simulink model "NatersV4_cleanV2"  (R2016a)
settings: Solver=FixedStepAuto  StartTime=1  StopTime=12*24*3  FixedStep=1  RelTol=1e-3
InitFcn:
  | %open the initialization function as a structure s
  | clear all
  | model = 'NatersV4_cleanV2';
  | s = system_init(model);
  | clear ans
  | 
  | % time vector
  | t=s.t;
  | t_step = t(2)-t(1);
  | time_u = s.time(1);
  | sample_time = s.sample_time;
  | 
  | % declare parameters
  | Text_D = s.Design(1);
  | Tin_D = s.Design(2);
  | Ts_D = s.Design(3);
  | Tr_D = s.Design(4);
  | Qdot_dem = s.Qdot_dem;
  | L_ini= s.L_ini;
  | 
  | Ab_c = s.Ab_c;
  | Bb_c = s.Bb_c;
  | Tin_sp = s.Tin_sp.signals.values;
  | Text = s.Text.signals.values;
  | Rad_90 = s.rad_90.signals.values;
  | 
  | % k parameters for heat pump model
  | K = s.k;
undefined symbols (not defined in the file or in its folder): DiscIntNeverNeededParam
libraries: simulink x20, carnot x2, dspsigops x1
(part 2 of 2)

== system NatersV4_cleanV2/Heat pump subsystem/cold side/Subsystem ==
  Tcold_out : Inport
  Abs : Abs
  Add : Sum  Inputs=-+
  Constant : Constant  Value=4
  PID Controller : simulink/Continuous/PID Controller  Controller=P  TimeDomain=Discrete-time  SampleTime=-1  IntegratorMethod=Forward Euler  FilterMethod=Forward Euler  Form=Parallel  UseFilter=on  ControllerParametersSource=internal  P=-0.5  I=1  D=0  N=100  InitialConditionSource=internal  InitialConditionForIntegrator=0  InitialConditionForFilter=0  ExternalReset=none  ZeroCross=off  LimitOutput=on  UpperSaturationLimit=1  LowerSaturationLimit=0  LinearizeAsGain=off  AntiWindupMode=none  Kb=1  TrackingMode=off  Kt=1  PParamMin=[]  PParamMax=[]  IParamMin=[]  IParamMax=[]  DParamMin=[]  DParamMax=[]  NParamMin=[]  NParamMax=[]  KbParamMin=[]  KbParamMax=[]  KtParamMin=[]  KtParamMax=[]  POutMin=[]  POutMax=[]  IOutMin=[]  IOutMax=[]  DOutMin=[]  DOutMax=[]  NOutMin=[]  NOutMax=[]  KbOutMin=[]  KbOutMax=[]  KtOutMin=[]  KtOutMax=[]  IntegratorOutMin=[]  IntegratorOutMax=[]  FilterOutMin=[]  FilterOutMax=[]  SumOutMin=[]  SumOutMax=[]  SumI1OutMin=[]  SumI1OutMax=[]  SumI2OutMin=[]  SumI2OutMax=[]  SumI3OutMin=[]  SumI3OutMax=[]  SumDOutMin=[]  SumDOutMax=[]  SaturationOutMin=[]  SaturationOutMax=[]  IntegratorContinuousStateAttributes=''  IntegratorStateMustResolveToSignalObject=off  IntegratorRTWStateStorageClass=Auto  FilterContinuousStateAttributes=''  FilterStateMustResolveToSignalObject=off  FilterRTWStateStorageClass=Auto  DifferentiatorICPrevScaledInput=0  DifferentiatorOutMin=[]  DifferentiatorOutMax=[]
  PID Controller1 : simulink/Continuous/PID Controller  Controller=PI  TimeDomain=Discrete-time  SampleTime=-1  IntegratorMethod=Backward Euler  FilterMethod=Forward Euler  Form=Parallel  UseFilter=on  ControllerParametersSource=internal  P=-0.8  I=-0.2/(60*sample_time)  D=0  N=100  InitialConditionSource=internal  InitialConditionForIntegrator=0  InitialConditionForFilter=0  ExternalReset=none  ZeroCross=off  LimitOutput=on  UpperSaturationLimit=1  LowerSaturationLimit=0  LinearizeAsGain=off  AntiWindupMode=back-calculation  Kb=1  TrackingMode=off  Kt=1  PParamMin=[]  PParamMax=[]  IParamMin=[]  IParamMax=[]  DParamMin=[]  DParamMax=[]  NParamMin=[]  NParamMax=[]  KbParamMin=[]  KbParamMax=[]  KtParamMin=[]  KtParamMax=[]  POutMin=[]  POutMax=[]  IOutMin=[]  IOutMax=[]  DOutMin=[]  DOutMax=[]  NOutMin=[]  NOutMax=[]  KbOutMin=[]  KbOutMax=[]  KtOutMin=[]  KtOutMax=[]  IntegratorOutMin=[]  IntegratorOutMax=[]  FilterOutMin=[]  FilterOutMax=[]  SumOutMin=[]  SumOutMax=[]  SumI1OutMin=[]  SumI1OutMax=[]  SumI2OutMin=[]  SumI2OutMax=[]  SumI3OutMin=[]  SumI3OutMax=[]  SumDOutMin=[]  SumDOutMax=[]  SaturationOutMin=[]  SaturationOutMax=[]  IntegratorContinuousStateAttributes=''  IntegratorStateMustResolveToSignalObject=off  IntegratorRTWStateStorageClass=Auto  FilterContinuousStateAttributes=''  FilterStateMustResolveToSignalObject=off  FilterRTWStateStorageClass=Auto  DifferentiatorICPrevScaledInput=0  DifferentiatorOutMin=[]  DifferentiatorOutMax=[]
  Saturation : Saturate  UpperLimit=1  LowerLimit=0  ZeroCross=off
  Scope{,1,3..4} (4 alike) : Scope
  Switch : Switch  Threshold=1.5
  control : Outport
  wires:
  Tcold_out/1 -> Add/1
  Add/1 -> Scope1/1, PID Controller/1, PID Controller1/1, Abs/1
  Abs/1 -> Switch/2
  PID Controller/1 -> Scope4/1, Switch/1
  PID Controller1/1 -> Switch/3, Scope3/1
  Switch/1 -> Saturation/1
  Constant/1 -> Add/2
  Saturation/1 -> control/1, Scope/1

== system NatersV4_cleanV2/Subsystem/Flow_Mixer_basic/Mix_T_Mdot ==
  THB1 : Inport
  THB2 : Inport  Port=2
  Add : Sum
  MATLAB Function : MATLAB Function  TreatAsAtomicUnit=on
  Scope : Scope
  Scope1 : Scope
  Selector1 : Selector  InputPortWidth=2  IndexOptions=Index vector (dialog)  Indices=[2]  OutputSizes=1
  Selector3 : Selector  InputPortWidth=2  IndexOptions=Index vector (dialog)  Indices=[2]  OutputSizes=1
  T : Outport
  mdot : Outport  Port=2
  wires:
  Add/1 -> mdot/1
  Selector1/1 -> Scope1/1, Add/2
  MATLAB Function/1(T_mix) -> T/1  "T"
  THB1/1 -> MATLAB Function/1(Flow_h), Selector3/1
  THB2/1 -> MATLAB Function/2(Flow_c), Selector1/1
  Selector3/1 -> Scope/1, Add/1

== matlab function NatersV4_cleanV2/Building subsystem/MATLAB Function ==
  data: Tb_in input size=[3 1]; Text input; Gin input; Psol input; Tb_out output size=[3 1]; Tws input; flow_fraction input; t_step parameter; time_u parameter; Qdem output size=1
function [Tb_out, Qdem]  = Simulate_building_dynamics(Tb_in , Text, Gin, Psol, Tws, flow_fraction,t_step, time_u)
%#codegen
% Twr   : Return temperature of the heating system
% Tf    : Temperature of floor
% Tr    : Temperature of the room

% state matrix x = [Twr, Tf, Tin]';
% input matrix u = [Text, Tws, Gin, Psol]'

[Ab_d, Bb_d,K_fr, K_wf,K_ra, C_wr, mc_f, thermal_capacity_flow] = get_state_input_mat_building(flow_fraction,t_step, time_u);

% F, L,
%Tws = 35;

%Tb_out = Ab_d * Tb_in + Bb_d * [Text; Qsup; Gin; Psol];
Tb_out = Ab_d * Tb_in + Bb_d * [Text; Tws; Gin; Psol];
%Qdem = K_fr * (Tb_out(2)-Tb_out(3));

% Qdem2 = K_fr * (Tb_in(1)-Tb_in(2));
Qdem = K_ra * (Tb_in(3)-Text)-Psol-Gin;
%Qdem = K_wf * (Tb_out(1)-Tb_out(2));
%Qsup = FH_st * mc_w * (Tws-Tb_out(1));
% Qsup = K_wf * (Tb_out(1)-Tb_out(2));
% Qin = mc_f * (Tb_in(2)-Tb_out(2))/(60/time_u*60);
% test = (Qdem + Qsup) - Qin;


function [Ab_d, Bb_d, K_fr,K_wf,K_ra, C_return, C_floor, thermal_capacity_flow, Qdot, facHP, nb] = get_state_input_mat_building(floor_heating_flow_fraction, t_step, time_u)

% Create the state matrix and the input matrix for the building system

% state vector for the building
% x_b = [Twr, Tf, Tin]'

% input vector for the building
% u_b = [Text, Tws, Qaux]



[C_return, C_floor, C_room, thermal_capacity_flow, K_wf, K_fr, K_ra, cp_w, Qdot] = get_param_building();
%mw_dot = thermal_capacity_flow * floor_heating_flow_fraction;
mw_dot = floor_heating_flow_fraction;

A = [...
[ -(K_wf + cp_w*mw_dot)/C_return,          K_wf/C_return,                     0];
[                   K_wf/C_floor, -(K_fr + K_wf)/C_floor,          K_fr/C_floor];
[                              0,            K_fr/C_room, -(K_fr + K_ra)/C_room] ...
];

B = [...
[           0, (cp_w*mw_dot)/C_return,        0,        0];
[           0,                      0,        0,        0];
[ K_ra/C_room,                      0, 1/C_room, 1/C_room] ...
];

if time_u == 24
    % time_unit = 'h';
    A = A.*3600;
    B = B.*3600;
elseif time_u == 4 % 1/4h
    A = A.*60*15;
    B = B.*60*15;
elseif time_u == 12 % 5 min
    A = A.*60*5;
    B = B.*60*5;
elseif time_u == 60 % 1 min
    A = A.*60;
    B = B.*60;  
elseif time_u == 60 % 1 min
    A = A.*1;
    B = B.*1;    
end

Ab_d = expm(t_step*A);
Bb_d = A\(Ab_d-eye(size(A, 1)))*B;


function [C_wr, mc_f, C_r, mdot_d_w, K_wf, K_fr, K_ra, cp_w, Q_D] = get_param_building()
%GET_PARAM_BUILDING returns the parameters of the selected building

cp_w = 4185;        % specific heat of water [J/kgK]
rho_w = 1000;       % density of water [kg/m3]
rho_air = 1.204;    % density of air [kg/m3]
V1 = 0.4;               % Volume of upper layer of storage tank [m3]
V2 = 0.4;               % Volume of middle layer of storage tank [m3]
V3 = 0.4;               % Volume of lower layer of storage tank [m3]
U_wf = 75;          % heat transfer coefficient of the distribution pipes [W/m2K] %48.2;
U_fr = 11.7;        % heat transfer coefficient between floor and room [W/m2K]
% \--> Source: On the heat transfer coefficients between heated/cooled radiant floorand room Tomasz Cholewaa
U_ra = 0.8;        % heat transfer coefficient of the wall [W/m2K] 1.19
A_fr = 350;         % floor surface [m2]
A_ra = 1080;         % wall surface [m2] 2*2.4H*(6l + 8L)=67.2
d_pipes = 0.033;   % internal diameter of the pipes [m]
d_dz = 0.2;        % space between the pipes [m]
L_pipes = A_fr/d_dz;    % length of the pipe [m]
A_wf = pi*d_pipes*L_pipes; % floor heating pipes surface [m2]
V_w = A_wf*d_pipes/4;      % Volume of water in distribution system [m3]0.228;
V_b = 6300;          % heated volume [m3]
K_wf = U_wf * A_wf; % thermal conductance of the distribution pipes [W/K]
K_fr = U_fr * A_fr; % thermal conductance between floor and room [W/K]
K_ra = U_ra * A_ra; % thermal conductance of the wall [W/K]
tau_r = 10;% 2.4
mc_f = 420e5;       % thermal capacity of the floor [J/K]

C_w = cp_w * rho_w * (V_w);%+V1+V2+V3);   % thermal capacity water [J/K]
%C_r = K_ra * tau_r;         % thermal capacity of the room [J/K]
C_r = V_b * rho_air * 1005 * tau_r; % thermal capacity of the room [J/K]
% Design hydronic system, rules Karlsson_and_Fahlen_2008
Text_D = -10;                   % Design outdoor temperature [K] 
Tin_D = 20;                     % Design outdoor temperature [K] 
Ts_D = 35;                      % Design supply temperature [K]  
Tr_D = 28;                      % Design return temperature [K]
Q_D = K_ra * (Tin_D - Text_D);  % Design heat demand [W]
mdot_d_w = Q_D / ((Ts_D - Tr_D)*cp_w);     % Design mass flow [kg/s]
v = mdot_d_w/(rho_w*(pi*(d_pipes^2)/4));   % Design velocity [m/s]
if v>1.2
    warning('The water velocity in the pipe is too high (noise"s problem are expected. Consider checking the diameter')
end
tau_HP =3*60;                   % Time constant Heat Pump [s]
C_ws = tau_HP * mdot_d_w * cp_w;           % thermal capacity supply water [J/K]
C_wr = C_w; %(C_w - C_ws)*10;        % thermal capacity return water [J/K]

== matlab function NatersV4_cleanV2/Subsystem/Flow_Mixer_basic/Mix_T_Mdot/MATLAB Function ==
  data: Flow_h input; Flow_c input; T_mix output size=[1]
function T_mix  = mix_temperature(Flow_h , Flow_c)

T1 = Flow_h(1);
T2 = Flow_c(1);

MDOT1 = Flow_h(2);
MDOT2 = Flow_c(2);
mdotsum = MDOT1+MDOT2;
NO_MASSFLOW = 0;
    
if mdotsum < NO_MASSFLOW      % if sum of massflows < limit: no massflow
    T_mix = 0.5*(T1+T2);        % average temperature 
elseif MDOT2 < NO_MASSFLOW    % else if massflow in path 2 < limit
    T_mix = T1;
elseif MDOT1 < NO_MASSFLOW   % else if massflow in path 1 < limit */
    T_mix = T2;
else                          % both pathes open */
    T_mix = (MDOT1*T1+MDOT2*T2)/mdotsum;
end
end

== matlab function NatersV4_cleanV2/Storage subsystem/MATLAB Function ==
  data: Ttes_in input double size=[3 1]; Tamb input; Twr input; Ttes_out output double size=[3 1]; Thp input; HP_st input; mdot_2_sto input; t_step parameter; time_u parameter; Qloss output
function [Ttes_out, Qloss]  = TES(Ttes_in, Tamb, Twr, Thp, HP_st, mdot_2_sto, t_step, time_u)
% coder.extrinsic('tic')
% coder.extrinsic('toc')
%coder.extrinsic('assignin')
%#codegen
% Tws   : Supply temperature of heating system (upper temperature of the storage tank)
% Tbb   : Lower temperature of the storage tank (return temperature of the HP)
% Thp_s : Supply temperature of the HP
% Twr   : Return temperature of the heating system

% state matrix x = [Tws, Tbm, Tbb]';
% input matrix u = [Tamb, Twr, Thp]'
%tic
[Ates_d, Btes_d, mc_w, K_sta_1, K_sta_2, K_sta_3] = get_state_input_mat_storage_test(HP_st, mdot_2_sto,t_step,time_u);
%toc
% F, L,

Ttes_out = Ates_d * Ttes_in + Btes_d * [Tamb; Twr; Thp];
%Qsup = FH_st*mc_w*(Ttes_out(1)-Ttes_out(2));
%Qsup1 = FH_st*mc_w*(Ttes_in(1)-Ttes_in(2));
Qloss= K_sta_1*(Ttes_in(1)-Tamb) + K_sta_2*(Ttes_in(2)-Tamb)+ K_sta_3*(Ttes_in(3)-Tamb);
%Qsup = FH_st*mc_w*(35-Twr);


%get_state_input_mat_storage(building_ID, HP_st, FH_st,t_step);
function [Ates_d, Btes_d, mc_w, K_sta_1, K_sta_2, K_sta_3] = get_state_input_mat_storage_test(HP_st, mdot_2_sto, t_step, time_u)
%%% The following lines allow to use specific function
%%% During simulation, the code generation software generates code for the call 
%%% to an extrinsic function, but does not generate the function's internal code
%%% !!!! CAREFULL it is much more slower !!!!
% coder.extrinsic('warning')
% coder.extrinsic('ss')
% coder.extrinsic('c2d')
% coder.extrinsic('ssdata')


% Create the state matrix and the input matrix for the thermal storage system

% state vector for the thermal storage
% x_b = [Tws, Tbm, Tbb]'

% input vector for the building
% u_b = [Text, Qhp, Qdem, Tset]

[C_tes_top, C_tes_mid, C_tes_bot, K_sta_1, K_sta_2, K_sta_3, K_l_12, K_l_23 , C_w_hp, C_w_fh, mc_w, cp_w, K_wa_fh, K_wa_hp] = get_param_storage_test();

% Matrix predefinition
nxb = 3;
nub = 3;

A = zeros(nxb,nxb); 
B = zeros(nxb,nub); 

F = HP_st; %'ToDo';

mc_hp = F * 0.68 * 4185;
mc_fh = mdot_2_sto * cp_w;
e=1;
 %% State Matrix
if mc_hp>mc_fh;
    % Equation for temperature of water supply Tws
    A(1,1) = -(mc_hp + K_sta_1 + K_l_12) / C_tes_top;
    A(1,2) = (K_l_12) / C_tes_top;

    % Equation for middle temperature of heating water buffer tank
    A(2,1) = ((mc_hp - mc_fh) + K_l_12) / C_tes_mid;
    A(2,2) = -((mc_hp - mc_fh) + K_sta_2 + K_l_12 + K_l_23) / C_tes_mid;
    A(2,3) = (K_l_23) / C_tes_mid;

    % Equation for bottom layers' temperature of heating water buffer tank
    A(3,2) = ((mc_hp - mc_fh) + K_l_23) / C_tes_bot;
    A(3,3) = - ((mc_hp - mc_fh) + mc_fh + K_sta_2 + K_l_23) / C_tes_bot;

    %% Input state matrix
    % input matrix u = [Tamb, Twr, Thp]'
    B(1,1) = K_sta_1 / C_tes_top;
    %B(1,2) = - mc_fh / C_tes_top;
    B(1,3) = mc_hp / C_tes_top; % 1/ C_tes_top;
    B(2,1) = K_sta_2 / C_tes_mid;
    B(3,1) = K_sta_3 / C_tes_bot;
    %if mc_fh ~= 0
    B(3,2) = mc_fh / C_tes_bot;
    %end
else
    % Equation for temperature of water supply Tws
    A(1,1) = -( mc_hp -(mc_hp - mc_fh) + K_sta_1 + K_l_12) / C_tes_top;
    A(1,2) = (-(mc_hp - mc_fh) + K_l_12) / C_tes_top;

    % Equation for middle temperature of heating water buffer tank
    A(2,1) = (K_l_12) / C_tes_mid;
    A(2,2) = -( -(mc_hp - mc_fh) + K_sta_2 + K_l_12 + K_l_23) / C_tes_mid;
    A(2,3) = (-(mc_hp - mc_fh) + K_l_23) / C_tes_mid;

    % Equation for bottom layers' temperature of heating water buffer tank
    A(3,2) = (K_l_23) / C_tes_bot;
    A(3,3) = - (mc_fh + K_sta_3 + K_l_23) / C_tes_bot;

    %% Input state matrix
    % input matrix u = [Tamb, Twr, Thp]'
    B(1,1) = K_sta_1 / C_tes_top;
    %B(1,3) = -mc_fh / C_tes_top;
    if mc_hp ~= 0
        B(1,3) = mc_hp / C_tes_top; % 1/ C_tes_top;
    end
    B(2,1) = K_sta_2 / C_tes_mid;
    B(3,1) = K_sta_3 / C_tes_bot;
    B(3,2) = mc_fh / C_tes_bot;
end

% B(3,1) = K_wa_hp / C_w_hp;
% B(3,3) = 1 / C_w_hp;

if time_u == 24
    % time_unit = 'h';
    A = A.*3600;
    B = B.*3600;
elseif time_u == 4 % 1/4h
    A = A.*60*15;
    B = B.*60*15;
elseif time_u == 12 % 5 min
    A = A.*60*5;
    B = B.*60*5;
elseif time_u == 60 % 1 min
    A = A.*60;
    B = B.*60;    
end

Ates_d = expm(t_step*A);
Btes_d = A\(Ates_d-eye(nxb))*B;

%%% !!!! CAREFULL it is much more slower !!!!
% sysb_c = ss(A, B, eye(nxb), zeros(nxb, size(B,2)));
% sysb_d = c2d(sysb_c, 1);
% [Ates_d, Btes_d] = ssdata(sysb_d);
% 
% stab_test = all(abs(eig(Ates_d))<1);
% if stab_test ~= 1
%     warning('The matrice A is not stable !!!')
% end
%%% !!!! CAREFULL it is much more slower !!!!



function [C_tes_top, C_tes_mid, C_tes_bot, K_sta_1, K_sta_2, K_sta_3, K_l_12, K_l_23 , C_w_hp, C_w_fh, mc_w, cp_w, K_wa_fh, K_wa_hp, C_sto] = get_param_storage_test()
%GET_PARAM_STORAGE returns the thermal storage parameters of the selected building
%building = ['Naters1', 'Naters2'];
%switch building(building_ID)
coder.extrinsic('assignin')
coder.extrinsic('matlab.lang.makeUniqueStrings')
%    case 'Naters1'
        cp_w = 4185;            % specific heat of water [J/kgK]
        rho_w = 1000;           % density of water [kg/m3]
        V1 = 0.4;               % Volume of upper layer of storage tank [m3]
        V2 = 0.4;               % Volume of middle layer of storage tank [m3]
        V3 = 0.4;               % Volume of lower layer of storage tank [m3] 
        V_w_hp = 0.1;           % Volume of water in distribution system (HP) [m3]
        V_w_fh = 0.188;         % Volume of water in distribution system (floor heating) [m3]0.128;
        Acs = 3.141;            % cross section storage tank [m2] 2*pi*r = pi (r=0.5)
        dz_1 = 0.63;            % height of upper layer [m]
        dz_2 = 0.63;            % height of middle layer [m]
        dz_3 = 0.63;            % height of lower layer [m]
        k_w = 0.65;             % thermal conductivity of water (at 20°C) [W/mK]
        U_wa = 11.7;            % heat transfer coefficient between floor and room [W/m2K]
        % \--> Source: On the heat transfer coefficients between heated/cooled radiant floorand room Tomasz Cholewaa
        U_sta = 0.7;            % heat transfer coefficient of the storage tank wall [W/m2K] % Source : CREM ALBI master thesis
        U_ra = 0.8;             % heat transfer coefficient of the wall [W/m2K] 1.86; (engineering toolbox 0.2 - 1.3 W/m2K) 
        A_wa_fh = 240;          % floor heating pipes surface [m2]
        L_hp = 10;              % pipes length HP to storage[m]
        A_ra = 1080;            % wall surface [m2] 2*2.4H*(6l + 8L)=67.2 326.4
        K_ra = U_ra * A_ra;     % thermal conductance of the wall [W/K]
        K_l_12 = Acs * k_w /(0.5 * (dz_1 + dz_2)); % thermal conductance between storage layers 1-2[W/K]
        K_l_23 = Acs * k_w /(0.5 * (dz_2 + dz_3)); % thermal conductance between storage layers 2-3[W/K]
        K_wa_fh = U_wa * A_wa_fh;     % thermal conductance of the distribution pipes (hp) [W/K]
        K_wa_hp = U_sta * L_hp;     % thermal conductance of the distribution pipes ([W/K]
        K_sta_1 = U_sta * Acs * dz_1; % thermal conductance between upper storage layer and outside [W/K]
        K_sta_2 = U_sta * Acs * dz_2; % thermal conductance between middle storage layer and outside [W/K]
        K_sta_3 = U_sta * Acs * dz_3; % thermal conductance between lower storage layer and outside [W/K]
%end
% dz =[dz_1 , dz_2, dz_3];
% Param_sto_n = repmat({'dz';'C_sto';'K_stamb'},1,4);
%Param_sto_n = matlab.lang.makeUniqueStrings(Param_sto_n(:,:));
% Param_sto_n(2,:) = {'C_sto'};
% Param_sto_n(3,:) = {'K_stamb'};
%Param_sto_n = matlab.lang.makeUniqueStrings(Param_sto_n{1,:});
% Param_sto = [dz_1/2, dz_2, dz_3*2;cp_w .* rho_w .* Acs .* dz; U_sta .* Acs .* dz];
% C_sto = cp_w .* rho_w .* Acs .* dz;
% K_stamb
% 
% for k =2:4
%     assignin('base',char(Param_sto_n{1,k}),Param_sto(1,k-1));
%     assignin('base',char(Param_sto_n{2,k}),Param_sto(2,k-1));
%     assignin('caller',char(Param_sto_n{3,k}),Param_sto(3,k-1));
%     %matlab.lang.makeUniqueStrings
% % C_tes_top = cp_w * rho_w * V1;  % thermal capacity of upper layer of storage [J/K]
% % C_tes_mid = cp_w * rho_w * V2;  % thermal capacity of middle layer of storage [J/K]
% % C_tes_bot = cp_w * rho_w * V3;  % thermal capacity of lower layer of storage [J/K]
% end


tau_HP =3*60;                   % Time constant Heat Pump [s]
C_tes_top = cp_w * rho_w * V1;  % thermal capacity of upper layer of storage [J/K]
C_tes_mid = cp_w * rho_w * V2;  % thermal capacity of middle layer of storage [J/K]
C_tes_bot = cp_w * rho_w * V3;  % thermal capacity of lower layer of storage [J/K]
C_w_hp = cp_w * rho_w * V_w_hp * tau_HP; % thermal capacity of water in distribution system (HP) [J/K]
C_w_fh = cp_w * rho_w * V_w_fh; % thermal capacity of water in distribution system (floor heating) [J/K]

% Design hydronic system, rules Karlsson_and_Fahlen_2008
Text_D = -10;                   % Design outdoor temperature [K] 
Tin_D = 20;                     % Design outdoor temperature [K] 
Ts_D = 35;                      % Design supply temperature [K]  
Tr_D = 28;                      % Design return temperature [K]
Q_D = K_ra * (Tin_D - Text_D);  % Design heat demand [W]
mc_w = Q_D / (Ts_D - Tr_D);     % Design thermal capacity flow [W/K]
C_ws = tau_HP * mc_w;           % thermal capacity supply water [J/K]
C_w_fh = C_w_fh - C_ws;              % thermal capacity return water [J/K]

== matlab function NatersV4_cleanV2/Storage subsystem/MATLAB Function1 ==
  data: Tsto_in input double size=[3 1]; Tamb input; Twr input; Ttes_out output double size=[3 1]; Thp input; HP_st input; mdot_2_sto input; Qloss output; sample_time input
function [Ttes_out, Qloss]  = TES_WORK_IN_PROGRESS_DO_NOT_DELETE(Tsto_in, Tamb, Twr, Thp, HP_st, mdot_2_sto, sample_time)

%#codegen
% Tws   : Supply temperature of heating system (upper temperature of the storage tank)
% Tbb   : Lower temperature of the storage tank (return temperature of the HP)
% Thp_s : Supply temperature of the HP
% Twr   : Return temperature of the heating system

% state matrix x = [Tsto1, sto1, ..., Tston]';
% u_b = [T_amb T_in1 T_in_2, ..., T_in_n]'


[A_sto_d, B_sto_d] = get_state_input_mat_storage(HP_st, mdot_2_sto,sample_time);


Ttes_out = A_sto_d * Tsto_in + B_sto_d * [Tamb; Twr; Thp];

%Qloss= K_sta_1*(Tsto_in(1)-Tamb) + K_sta_2*(Tsto_in(2)-Tamb)+ K_sta_3*(Ttes_in(3)-Tamb);

[cp_w, rho_w, kv] = water_property(Ttes_in');


%get_state_input_mat_storage(building_ID, HP_st, FH_st,t_step);
function [A_sto_d, B_sto_d, mc_w, K_sta_1, K_sta_2, K_sta_3] = get_state_input_mat_storage(HP_st, mdot_2_sto, sample_time)
% Create the state matrix and the input matrix for the thermal storage system

% state vector for the thermal storage. 1 is the top layer and n is the bottom
% x_b = [T_sto1, T_sto2,..., T_ston]'

% input vector for the building
% u_b = [T_amb T_in1 T_in_2, ..., T_in_n]
% T_in_i represents the input temperature of the different fluid entering the storage tank

%% Geometry
cp_w = [4185 4185 4185 4185 4185 4185];
rho_w = [1000 1000 1000 1000 1000 1000];
kv = [0.65 0.65 0.65 0.65 0.65 0.65];
nb_nodes = 6;
nb_loops = 3;
V_sto = 1.2;            % Volume of storage tank [m3]
h_sto = 2;              % Height of storage tank [m]
Acs = V_sto / h_sto;    % cross section storage tank [m2]
loop_in_out = [ 1 6 ; 5 2 ; 3 5];
if max(loop_in_out) > nb_nodes
    warning('The number of nodes and the input position of the fluid loops are not consistent !!')
end
if size(loop_in_out,1) > nb_loops
    warning('The number of loops and the input position of the fluid loops are not consistent !!')
end
[loop_in_pos, ind] = sort(loop_in_out(:,1)');
nb_mix_up = min(min(loop_in_out))-1;
nb_mix_bot = nb_nodes-max(max(loop_in_out));
nb_nodes_cor = nb_nodes - nb_mix_up - nb_mix_bot;
dz= h_sto*ones(1,nb_nodes_cor)/nb_nodes_cor;        % layer height [m]

U_sta = 0.7;                        % heat transfer coefficient of the storage tank wall [W/m2K] % Source : CREM ALBI master thesis
K_stamb =  U_sta * Acs * dz(1);     % thermal conductance between storage layer i and outside [W/K]
C_sto = cp_w .* rho_w .* Acs .* dz(1); % thermal capacity of storage layer i [J/K]
m_dot = [0.68, 0.5, 0.6];
mcp_dot_in = cp_w_in.*m_dot;
sign_flow = zeros(1,nb_loops);
flow_geom = zeros(nb_nodes_cor-1, nb_loops); % sparse

for j = 1:nb_loops
    sign_flow(j) = -sign(loop_in_out(j,1)-loop_in_out(j,2));
    flow_geom(min(loop_in_out(j,:)):max(loop_in_out(j,:))-1,j) =sign_flow(j);
end
mcp_dot_sto_n = cp_w.*flow_geom*m_dot';
alpha = (sign(mcp_dot_sto_n)<=0)==0;

%% Matrix definition
A_sto = zeros(nb_nodes_cor,nb_nodes_cor);
B_sto = zeros(nb_nodes_cor,nb_loops+1);
idx = sub2ind(size(B_sto), loop_in_pos, 1+ind); % index of position of the flow entry in the storage tank
B_sto(idx) = mcp_dot_in(ind)/C_sto;

for i =2+nb_mix_up:nb_nodes-1-nb_mix_bot
    A_sto(1,1:2) = [((1-alpha(1)) * mcp_dot_sto_n(1) - kv(1) * Acs * (1 / (0.5 * dz(1))) - K_stamb) / C_sto(1), (- (1 - alpha(1)) * mcp_dot_sto_n(1) + kv(1) * Acs * (1 / (0.5 * dz(1)))) / C_sto(1)];
    A_sto(i,i-1:i+1) = [(alpha(i-1) * mcp_dot_sto_n(i-1) + kv(i) * Acs * (1 / (0.5 * dz(i-1)))) / C_sto(i), (- alpha(i-1) * mcp_dot_sto_n(i-1) + (1-alpha(i)) * mcp_dot_sto_n(i) - K_stamb - kv(i) * Acs * (1 /(0.5 * dz(i-1)) + 1 / (0.5 * dz(i)))) / C_sto(i), ((1-alpha(i)) * mcp_dot_sto_n(i) + kv(i) * Acs * (1 / 0.5 * dz(i)))/C_sto(i)];
    A_sto(end,end-1:end) = [((alpha(end)) * mcp_dot_sto_n(end) - kv(end) * Acs * (1 / (0.5 * dz(end)))) / C_sto(end), (- alpha(end) * mcp_dot_sto_n(end) - K_stamb + kv(end) * Acs * (1 / (0.5 * dz(end)))) / C_sto(end)];
  
    B_sto(i-1:end,1) = K_stamb/ C_sto;
end


 %% State Matrix

A_sto = A_sto.*sample_time;
B_sto = B_sto.*sample_time;

A_sto_d = expm(t_step*A_sto);
B_sto_d = A_sto\(A_sto_d-eye(nxb))*B_sto;


function [cp_w, rho_w, kv] = water_property(T_w)
w_prop_mat = [0 35 70; 4217.6, 4174, 4189.5; 999.8 993.5 977.8]; % [T;cp;rho]  

% SOURCE: New International Formulation for the Thermal Conductivity of H2O
% Coefficients ci and di in Eq.(21) for the thermal conductivity of liquid water at 0.1 MPa.
ci = [1.663, -1.778, 1.1567, -0.432115];
di = [-1.15, -3.4, -6, -7.6];
kv=zeros(1,length(T_w));
cp_w=zeros(1,length(T_w));
rho_w=zeros(1,length(T_w));
for i=1:length(T_w)
    if i<length(T_w)
        kv(i) = ci*((273.15 + (T_w(i)+T_w(i+1))/2)/300).^(di)'; % thermal conductivity of water (0.65 at 20°C) [W/mK]
    end
    if T_w(i) <= w_prop_mat(1,2)
        cp_w(i) = ((w_prop_mat(2,2)-w_prop_mat(2,1))*(T_w(i)-w_prop_mat(1,1)))/(w_prop_mat(1,2)-w_prop_mat(1,1)) + w_prop_mat(2,1);  % specific heat of water [J/kgK]
        rho_w(i) = ((w_prop_mat(3,2)-w_prop_mat(3,1))*(T_w(i)-w_prop_mat(1,1)))/(w_prop_mat(1,2)-w_prop_mat(1,1)) + w_prop_mat(3,1); % density of water [kg/m3]
    else
        cp_w(i) = ((w_prop_mat(2,3)-w_prop_mat(2,2))*(T_w(i)-w_prop_mat(1,2)))/(w_prop_mat(1,3)-w_prop_mat(1,2)) + w_prop_mat(2,2);  % specific heat of water [J/kgK]
        rho_w(i) = ((w_prop_mat(3,3)-w_prop_mat(3,2))*(T_w(i)-w_prop_mat(1,2)))/(w_prop_mat(1,3)-w_prop_mat(1,2)) + w_prop_mat(3,2); % density of water [kg/m3]
    end
end
